simulink model "flc_simulink_file"  (R2023a)
settings: Solver=FixedStepAuto  StartTime=0.0  StopTime=0.18  MaxStep=5.0E-7  RelTol=1e-3  EnableMultiTasking=on
undefined symbols (not defined in the file): Acid, Lead
libraries: spsSeriesRLCBranchLib x3, spsBatteryLib x1, spsCurrentMeasurementLib x1, spsDiodeLib x1, fuzblock x1, spsIGBTDiodeLib x1, spsPVArrayLib x1, spsPWMGeneratorDCDCLib x1, spsVoltageMeasurementLib x1, spspowerguiLib x1
settings Model: Creator=SEIL  LastModifiedBy=SEIL
settings OptimizationCC: EnhancedBackFolding=on  PassReuseOutputArgsAs=Individual arguments  ZeroExternalMemoryAtStartup=off  ZeroInternalMemoryAtStartup=off  MaxStackSize=64  OptimizeBlockOrder=speed  DifferentSizesBufferReuse=on  OptimizationCustomize=off  EfficientTunableParamExpr=on
settings DebuggingCC: ParameterTunabilityLossMsg=error  SFcnCompatibilityMsg=warning  SFUnexpectedBacktrackingDiag=warning  SFNoUnconditionalDefaultTransitionDiag=warning
settings HardwareCC: ProdBitPerPointer=32  ProdBitPerSizeT=32  ProdBitPerPtrDiffT=32  ProdLargestAtomicInteger=Long  ProdLargestAtomicFloat=Double  ProdWordSize=32  ProdLongLongMode=on  ProdHWDeviceType=ARM Compatible->ARM Cortex  TargetBitPerPointer=64  TargetBitPerSizeT=64  TargetBitPerPtrDiffT=64  TargetLongLongMode=on  TargetIntDivRoundTo=Zero  TargetEndianess=LittleEndian  TargetWordSize=64  TargetHWDeviceType=MATLAB Host  ProdEqTarget=off
settings SFSimCC: MATLABDynamicMemAlloc=off
settings RTWCC: Description=Embedded Coder  SystemTargetFile=ert.tlc  HardwareBoard=STM32G4xx Based  TemplateMakefile=ert_default_tmf  GenerateReport=on  Toolchain=GNU Tools for ARM Embedded Processors  BuildConfiguration=Debug  LaunchReport=on  CheckMdlBeforeBuild=Warning
settings CodeAppCC: ForceParamTrailComments=on  IgnoreCustomStorageClasses=off  OperatorAnnotations=on  SimulinkDataObjDesc=on  SFDataObjDesc=on  InsertBlockDesc=on  EnableCustomComments=on
settings ERTTargetCC: CodeReplacementLibrary=ARM Cortex-M  ExtModeTransport=3  ExtModeStaticAlloc=on  ExtModeStaticAllocSize=2048  ExtModeMexFile=ext_xcp  ExtModeIntrfLevel=Level2 - Open
settings ConfigComp: DVTestSuiteOptimization=Auto  DVDetectOutOfBounds=on  DVModelReferenceHarness=on  DVHarnessSource=Signal Editor

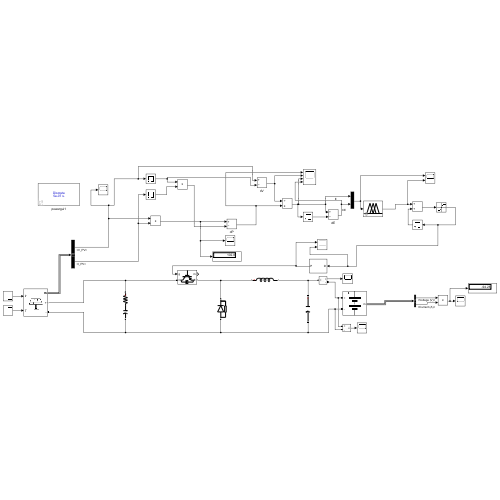
[thumbnail: Simulink's stored preview of the top-level diagram]
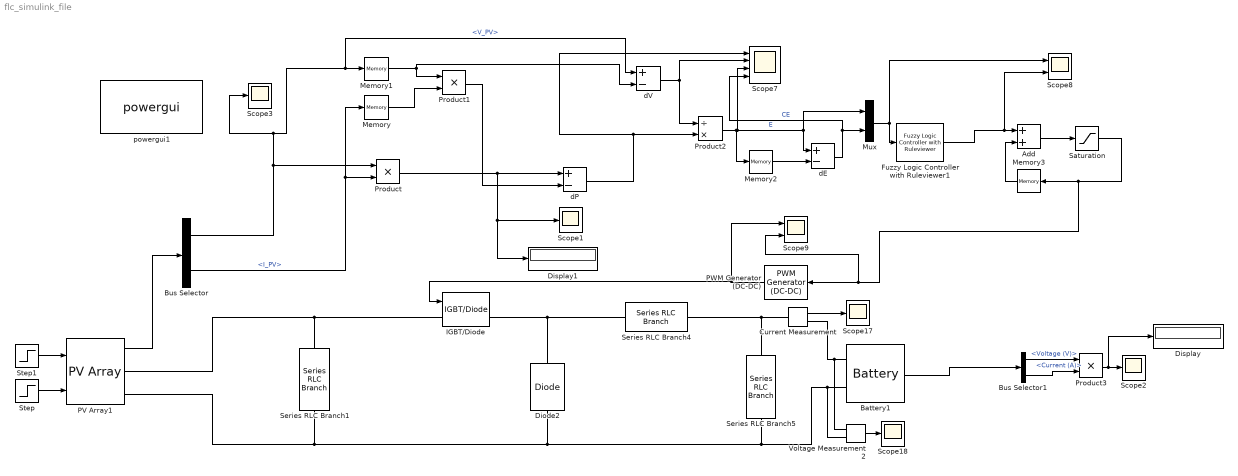
== system flc_simulink_file ==
  Add : Sum
  Battery1 : spsBatteryLib/Battery  BatType=Lead-Acid  ShowTempParam=off  ThermalPreset=no  ShowAgeParam=off  NomV=12  NomQ=500  SOC=0  Batt_Tr=0.01  PresetModel=on  MaxQ=520.8333  MinV=9  FullV=13.0658  Dis_rate=100  R=0.00024  Normal_OP=155.1389  expZone="[12.2171      1.66667]"  current=[6.5 13 32.5]  Units=Time  Tci=20  NomT=20  T2=-30  MaxQ2=4.8  FullV2=7.1  Normal_OP2=5.655  expZone2="[6.58           1]"  Rca=0.6  ti=2000  Dp=0  Neq0=0  Tsim=1e6  Ta1=25  Qeol=5.4*0.9  Reol=0.013333*1.2  Char_age=[2.3478, 3]  Dis_age=[2.3478, 10]  N1=1500  N2=10500  N3=1000  N4=1400  Ta2=45  N5=950
  Bus Selector : BusSelector  OutputSignals=V_PV,I_PV
  Bus Selector1 : BusSelector  OutputSignals=Voltage (V),Current (A)
  Current Measurement : spsCurrentMeasurementLib/Current Measurement  PhasorSimulation=off  OutputType=Complex  PSBequivalent=0
  Diode2 : spsDiodeLib/Diode  Ron=0.001  Lon=0  Vf=0.8  IC=0  UseSnubber=0  Rs=500  Cs=250e-9  Measurements=off
  Display : Display
  Display1 : Display
  Fuzzy Logic Controller with Ruleviewer1 : fuzblock/Fuzzy Logic  Controller  with Ruleviewer  fismatrix=fis  Ts=2
  IGBT/Diode : spsIGBTDiodeLib/IGBT//Diode  Ron=1e-3  Rs=1e5  Cs=inf  Measurements=on
  Memory{,1..3} (4 alike) : Memory  InheritSampleTime=on
  Mux : Mux  Inputs=2
  PV Array1 : spsPVArrayLib/PV Array  Npar=1  Nser=1  PlotType=one module @ 25 deg.C & specified irradiances  S_vec="[ 1000  500  100 ]"  Temp_C_vec="[ 45 25  ]"  ModuleName=A2Peak Power POWER ON P220-6x10  PlotWhenSelected=off  Pm=219.978  Ncell=60  Voc=36.72  Isc=7.98  Vm=30.3  Im=7.26  beta_Voc_pc=-0.35  alpha_Isc_pc=0.05  beta_Voc=-0.12852  alpha_Isc=0.00399  IL=8.0041  I0=1.8441e-10  nI=0.97472  Rsh=85.0716  Rs=0.25728  RobustModel=off  RobustCellTemperature=313.3991  BAL=on  Tc=1e-6  Tfilter=5e-5
  PWM Generator (DC-DC) : spsPWMGeneratorDCDCLib/PWM Generator (DC-DC)  Fsw=10000  Ts=0
  Product : Product
  Product1 : Product
  Product2 : Product  Inputs=/*
  Product3 : Product
  Saturation : Saturate  UpperLimit=0.92  LowerLimit=0
  Scope{1..3,17..18} (5 alike) : Scope
  Scope7 : Scope  NumInputPorts=4
  Scope8 : Scope  NumInputPorts=2
  Scope9 : Scope  NumInputPorts=2
  Series RLC Branch1 : spsSeriesRLCBranchLib/Series RLC Branch  LConnTagsString=__new0  RConnTagsString=__new0  BranchType=RC  Resistance=0.001  Inductance=0  SetiL0=off  InitialCurrent=0  Capacitance=1000e-6  Setx0=off  InitialVoltage=0  Measurements=None
  Series RLC Branch4 : spsSeriesRLCBranchLib/Series RLC Branch  LConnTagsString=__new0  RConnTagsString=__new0  BranchType=L  Resistance=1  Inductance=0.8653e-3  SetiL0=off  InitialCurrent=0  Capacitance=1e-6  Setx0=off  InitialVoltage=0  Measurements=None
  Series RLC Branch5 : spsSeriesRLCBranchLib/Series RLC Branch  LConnTagsString=__new0  RConnTagsString=__new0  BranchType=C  Resistance=1  Inductance=1e-3  SetiL0=off  InitialCurrent=0  Capacitance=369.79e-6  Setx0=off  InitialVoltage=0  Measurements=None
  Step : Step  Time=0.03  Before=25  After=40  SampleTime=0
  Step1 : Step  Time=0.04  Before=1000  After=500  SampleTime=0
  Voltage Measurement2 : spsVoltageMeasurementLib/Voltage Measurement  PhasorSimulation=off  OutputType=Complex  PSBequivalent=0
  dE : Sum  Inputs=+-
  dP : Sum  Inputs=+-
  dV : Sum  Inputs=+-
  powergui1 : spspowerguiLib/powergui  Priority=1  SimulationMode=Discrete  SampleTime=50e-8  frequency=60  Iterations=50  frequencyindice=0  Pbase=100e6  ErrMax=1e-4  UnitsV=kV  UnitsW=MW  buscounter=0  FunctionMessages=off  echomessages=off  EnableUseOfTLC=off  CurrentSourceSwitches=off  DisableSnubberDevices=off  DisableRonSwitches=off  DisableVfSwitches=off  DisplayEquations=off  AutomaticDiscreteSolvers=off  SolverType=Tustin/Backward Euler (TBE)  Interpol=off  ExternalGateDelay=off  methode=off  Ts=100  x0status=blocks  SPID=on  SwTol=0  HookPort=off  NonlinearTolerance=1e-4  nMaxIteration=100  ContinueOnMaxIteration=off  RestoreLinks=warning  ResistiveCurrentMeasurement=off  Frange=[0:2:500]  Ylog=off  Xlog=on  ShowGrid=off  save=off  variable=ZData  structure=0  ZoomFFT=off  StartTime=0.0  cycles=1  DisplayStyle=1  fundamental=60  FreqAxis=off  MaxFrequency=1000  frequencyindicesteady=1  RmsSteady=1  display=off
  wires:
  Bus Selector/1 -> Product/1, Memory1/1, dV/1, Scope3/1  "<V_PV>"
  Bus Selector/2 -> Product/2, Memory/1  "<I_PV>"
  Memory1/1 -> dV/2, Product1/1
  Memory/1 -> Product1/2
  Product/1 -> Scope1/1, Display1/1, dP/1
  dV/1 -> Scope7/2, Product2/1
  dP/1 -> Product2/2, Scope7/1
  Product2/1 -> Scope7/3, Mux/1, dE/1, Memory2/1  "E"
  Memory2/1 -> dE/2
  dE/1 -> Scope7/4, Mux/2  "CE"
  Add/1 -> Saturation/1
  Memory3/1 -> Add/2
  Bus Selector1/1 -> Product3/1  "<Voltage (V)>"
  Bus Selector1/2 -> Product3/2  "<Current (A)>"
  Product3/1 -> Display/1, Scope2/1
  Battery1/1 -> Bus Selector1/1
  PWM Generator (DC-DC)/1 -> IGBT/Diode/1, Scope9/1
  PV Array1/1 -> Bus Selector/1
  Mux/1 -> Fuzzy Logic Controller with Ruleviewer1/1, Scope8/1
  Product1/1 -> dP/2
  Fuzzy Logic Controller with Ruleviewer1/1 -> Scope8/2, Add/1
  Current Measurement/1 -> Scope17/1
  Voltage Measurement2/1 -> Scope18/1
  Saturation/1 -> Memory3/1, Scope9/2, PWM Generator (DC-DC)/1
  Step/1 -> PV Array1/2
  Step1/1 -> PV Array1/1
  connections:
  Diode2/RConn1 -- Series RLC Branch4/LConn1 -- IGBT/Diode/RConn1
  Diode2/LConn1 -- Series RLC Branch5/RConn1 -- Voltage Measurement2/LConn2 -- Battery1/LConn2 -- PV Array1/RConn2 -- Series RLC Branch1/RConn1
  Series RLC Branch4/RConn1 -- Current Measurement/LConn1 -- Series RLC Branch5/LConn1
  IGBT/Diode/LConn1 -- Series RLC Branch1/LConn1 -- PV Array1/RConn1
  Current Measurement/RConn1 -- Voltage Measurement2/LConn1 -- Battery1/LConn1
